simulink subsystem "no_reg_frame_ctrl"  (R2019b)
settings: Solver=VariableStepAuto  StartTime=0.0  StopTime=10.0  RelTol=1e-3
settings Model: Creator=torha  LastModifiedBy=torha

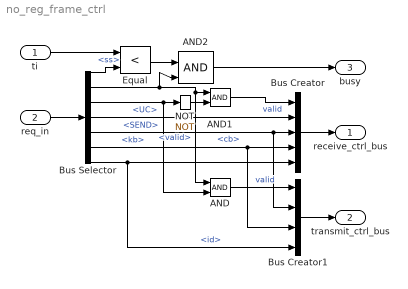
== system no_reg_frame_ctrl ==
  ti : Inport
  req_in : Inport  Port=2
  AND : Logic  IconShape=distinctive  AllPortsSameDT=off  OutDataTypeStr=boolean
  AND1 : Logic  IconShape=distinctive  AllPortsSameDT=off  OutDataTypeStr=boolean
  AND2 : Logic  IconShape=distinctive  AllPortsSameDT=off  OutDataTypeStr=boolean
  Bus Creator : BusCreator  Inputs=5
  Bus Creator1 : BusCreator  Inputs=4
  Bus Selector : BusSelector  OutputSignals=req.ss,valid,req.SEND,req.UC,req.cb,req.kb,id
  Equal : RelationalOperator  Operator=<  OutDataTypeStr=boolean  RndMeth=Simplest
  NOT : Logic  Operator=NOT  IconShape=distinctive  AllPortsSameDT=off  OutDataTypeStr=boolean
  receive_ctrl_bus : Outport
  transmit_ctrl_bus : Outport  Port=2
  busy : Outport  Port=3
  wires:
  req_in/1 -> Bus Selector/1
  ti/1 -> Equal/1
  Bus Creator/1 -> receive_ctrl_bus/1
  Bus Creator1/1 -> transmit_ctrl_bus/1
  AND/1 -> Bus Creator1/1  "valid"
  AND1/1 -> Bus Creator/1  "valid"
  NOT/1 -> AND1/2
  Bus Selector/6 -> Bus Creator/4, Bus Creator1/3  "<kb>"
  Bus Selector/1 -> Equal/2  "<ss>"
  Bus Selector/3 -> AND/2, NOT/1  "<SEND>"
  Bus Selector/4 -> Bus Creator/2  "<UC>"
  Bus Selector/5 -> Bus Creator/3, Bus Creator1/2  "<cb>"
  Bus Selector/2 -> AND1/1, AND/1, AND2/2  "<valid>"
  Equal/1 -> AND2/1
  AND2/1 -> busy/1
  Bus Selector/7 -> Bus Creator/5, Bus Creator1/4  "<id>"
